simulink model "lab4_prep"  (R2022a)
settings: Solver=VariableStepAuto  StartTime=0.0  StopTime=30.0  RelTol=10e-10  AbsTol=10e-10
values from neighbouring files (symbols this model uses):
  Actrl = A + B*K_ctrl-L_ctrl*C    [lab4.m]
  Bctrl = [L_ctrl,-B*K_ctrl]    [lab4.m]
  C = [1 0 0 0; 0 0 1 0]    [lab4.m]
  Cctrl = K_ctrl    [lab4.m]
  Dctrl = [0,0,-K_ctrl]    [lab4.m]
  K_sfs = K_ctrl    [lab4.m]
  Ulim = 5.875    [lab4.m]
  x0 = [0; 0; pi/24; 0]    [lab4.m]
settings Model: Creator=sun  LastModifiedBy=yuans
settings ModelReferenceCC: EnableRefExpFcnMdlSchedulingChecks=off
settings RTWCC: Description=Generic Real-Time Target  GPUComputeCapability=5.0

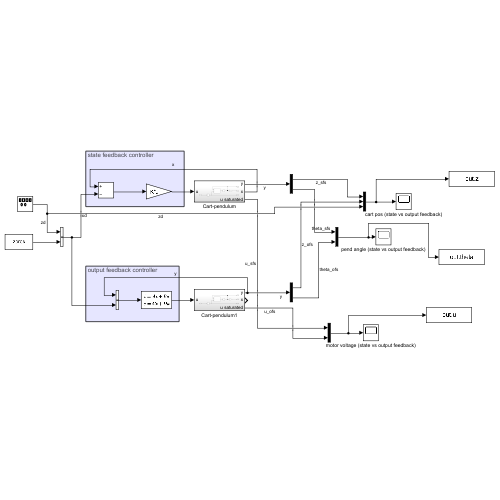
[thumbnail: Simulink's stored preview of the top-level diagram]
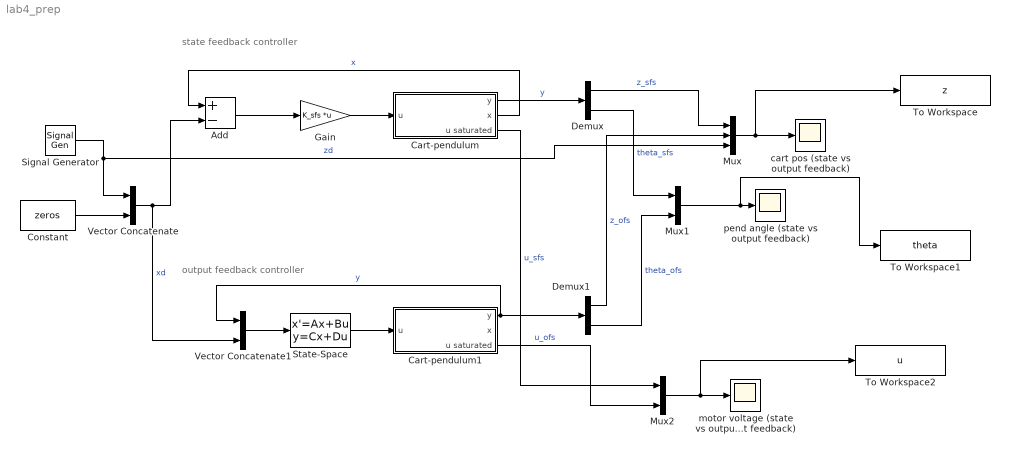
== system lab4_prep ==
  note: state feedback controller
  note: output feedback controller
  Add : Sum  Inputs=+-
  Cart-pendulum : Subsystem
  Cart-pendulum1 : Subsystem
  Constant : Constant  Value=zeros
  Demux : Demux  Outputs=2
  Demux1 : Demux  Outputs=2
  Gain : Gain  Gain=K_sfs  Multiplication=Matrix(K*u)
  Mux : Mux  Inputs=3
  Mux1 : Mux  Inputs=2
  Mux2 : Mux  Inputs=2
  Signal Generator : SignalGenerator  WaveForm=square  Amplitude=0.1  Frequency=0.1
  State-Space : StateSpace  A=Actrl  B=Bctrl  C=Cctrl  D=Dctrl  InitialCondition=0
  To Workspace : ToWorkspace  VariableName=z  SaveFormat=Timeseries  SampleTime=-1
  To Workspace1 : ToWorkspace  VariableName=theta  SaveFormat=Timeseries  SampleTime=-1
  To Workspace2 : ToWorkspace  VariableName=u  SaveFormat=Timeseries  SampleTime=-1
  Vector Concatenate : Concatenate
  Vector Concatenate1 : Concatenate
  cart pos (state vs output feedback) : Scope
  motor voltage (state vs output feedback) : Scope
  pend angle (state vs output feedback) : Scope
  wires:
  Constant/1 -> Vector Concatenate/2
  Signal Generator/1 -> Mux/3, Vector Concatenate/1  "zd"
  Gain/1 -> Cart-pendulum/1(u)
  Add/1 -> Gain/1
  Vector Concatenate/1 -> Vector Concatenate1/2, Add/2  "xd"
  Cart-pendulum/2(x) -> Add/1  "x"
  Cart-pendulum1/1(y) -> Vector Concatenate1/1, Demux1/1  "y"
  Cart-pendulum/1(y) -> Demux/1  "y"
  Demux/1 -> Mux/1  "z_sfs"
  Demux/2 -> Mux1/1  "theta_sfs"
  Demux1/1 -> Mux/2  "z_ofs"
  Demux1/2 -> Mux1/2  "theta_ofs"
  Cart-pendulum/3(u saturated) -> Mux2/1  "u_sfs"
  Cart-pendulum1/3(u saturated) -> Mux2/2  "u_ofs"
  Mux2/1 -> To Workspace2/1, motor voltage (state vs output feedback)/1
  Mux1/1 -> To Workspace1/1, pend angle (state vs output feedback)/1
  Mux/1 -> To Workspace/1, cart pos (state vs output feedback)/1
  Vector Concatenate1/1 -> State-Space/1
  State-Space/1 -> Cart-pendulum1/1(u)

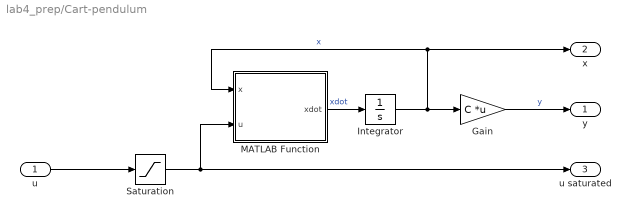
== system lab4_prep/Cart-pendulum ==
  u : Inport
  Gain : Gain  Gain=C  Multiplication=Matrix(K*u)
  Integrator : Integrator  InitialCondition=x0
  MATLAB Function : MATLAB Function  TreatAsAtomicUnit=on
  Saturation : Saturate  UpperLimit=Ulim  LowerLimit=-Ulim
  y : Outport
  x : Outport  Port=2
  u saturated : Outport  Port=3
  wires:
  MATLAB Function/1(xdot) -> Integrator/1  "xdot"
  u/1 -> Saturation/1
  Integrator/1 -> x/1, MATLAB Function/1(x), Gain/1  "x"
  Saturation/1 -> u saturated/1, MATLAB Function/2(u)
  Gain/1 -> y/1  "y"

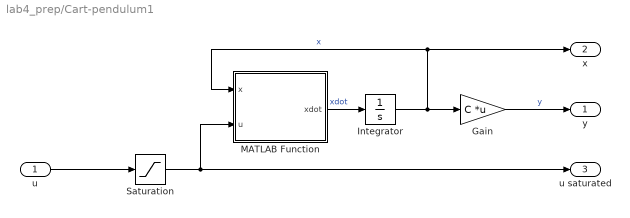
== system lab4_prep/Cart-pendulum1 ==
  u : Inport
  Gain : Gain  Gain=C  Multiplication=Matrix(K*u)
  Integrator : Integrator  InitialCondition=x0
  MATLAB Function : MATLAB Function  TreatAsAtomicUnit=on
  Saturation : Saturate  UpperLimit=Ulim  LowerLimit=-Ulim
  y : Outport
  x : Outport  Port=2
  u saturated : Outport  Port=3
  wires:
  MATLAB Function/1(xdot) -> Integrator/1  "xdot"
  u/1 -> Saturation/1
  Integrator/1 -> x/1, MATLAB Function/1(x), Gain/1  "x"
  Saturation/1 -> u saturated/1, MATLAB Function/2(u)
  Gain/1 -> y/1  "y"

== matlab function lab4_prep/Cart-pendulum/MATLAB Function ==
  data: x input; u input; xdot output
function xdot = cartpend(x,u)

xdot = cartpend(x,u);

== matlab function lab4_prep/Cart-pendulum1/MATLAB Function ==
  data: x input; u input; xdot output
function xdot = cartpend(x,u)

xdot = cartpend(x,u);
